simulink model "Simulation_Sprungantwort"  (R2019a)
settings: Solver=FixedStepAuto  StartTime=0.0  StopTime=12  FixedStep=1/1e4  RelTol=1e-3
settings Model: Creator=basti  LastModifiedBy=aaron
settings DebuggingCC: SFMachineParentedDataDiag=error

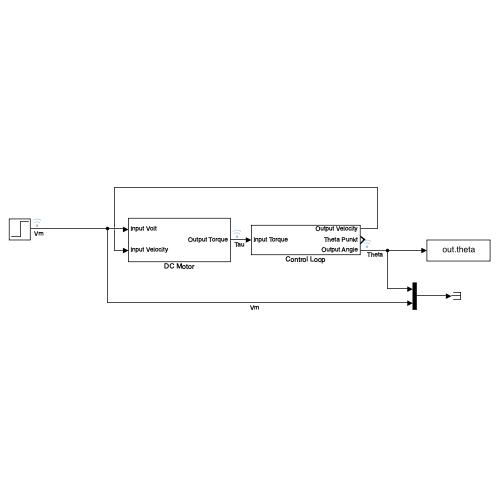
[thumbnail: Simulink's stored preview of the top-level diagram]
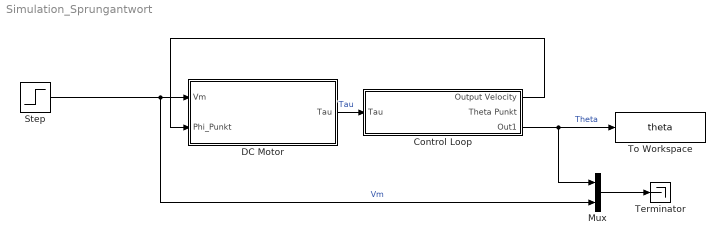
== system Simulation_Sprungantwort ==
  Control Loop : Subsystem
  DC Motor : Subsystem
  Mux : Mux  Inputs=2
  Step : Step  Time=0.5  After=[10 15 20]  SampleTime=0
  Terminator : Terminator
  To Workspace : ToWorkspace  VariableName=theta  SampleTime=-1
  wires:
  DC Motor/1(Tau) -> Control Loop/1(Tau)  "Tau"
  Control Loop/1(Output Velocity) -> DC Motor/2(Phi_Punkt)
  Control Loop/3(Out1) -> To Workspace/1, Mux/1  "Theta"
  Mux/1 -> Terminator/1
  Step/1 -> Mux/2, DC Motor/1(Vm)  "Vm"

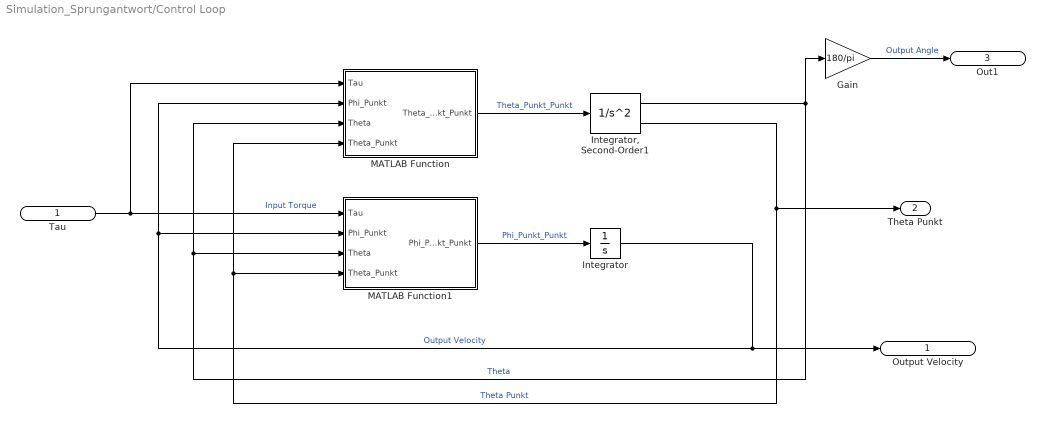
== system Simulation_Sprungantwort/Control Loop ==
  Tau : Inport
  Gain : Gain  Gain=180/pi
  Integrator : Integrator
  "Integrator, Second-Order1" : SecondOrderIntegrator  ICX=pi
  MATLAB Function : MATLAB Function  TreatAsAtomicUnit=on
  MATLAB Function1 : MATLAB Function  TreatAsAtomicUnit=on
  Output Velocity : Outport
  Theta Punkt : Outport  Port=2
  Out1 : Outport  Port=3
  wires:
  MATLAB Function/1(Theta_Punkt_Punkt) -> "Integrator, Second-Order1"/1  "Theta_Punkt_Punkt"
  MATLAB Function1/1(Phi_Punkt_Punkt) -> Integrator/1  "Phi_Punkt_Punkt"
  Integrator/1 -> Output Velocity/1, MATLAB Function1/2(Phi_Punkt), MATLAB Function/2(Phi_Punkt)  "Output Velocity"
  "Integrator, Second-Order1"/1 -> MATLAB Function1/3(Theta), MATLAB Function/3(Theta), Gain/1  "Theta"
  "Integrator, Second-Order1"/2 -> Theta Punkt/1, MATLAB Function/4(Theta_Punkt), MATLAB Function1/4(Theta_Punkt)  "Theta Punkt"
  Tau/1 -> MATLAB Function/1(Tau), MATLAB Function1/1(Tau)  "Input Torque"
  Gain/1 -> Out1/1  "Output Angle"

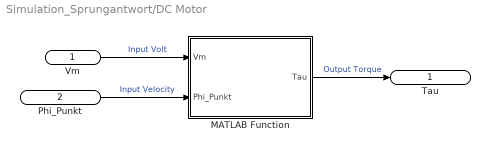
== system Simulation_Sprungantwort/DC Motor ==
  Vm : Inport
  Phi_Punkt : Inport  Port=2
  MATLAB Function : MATLAB Function  TreatAsAtomicUnit=on
  Tau : Outport
  wires:
  Vm/1 -> MATLAB Function/1(Vm)  "Input Volt"
  Phi_Punkt/1 -> MATLAB Function/2(Phi_Punkt)  "Input Velocity"
  MATLAB Function/1(Tau) -> Tau/1  "Output Torque"

== matlab function Simulation_Sprungantwort/Control Loop/MATLAB Function1 ==
  data: Tau input; Phi_Punkt_Punkt output; Phi_Punkt input; Theta input; Theta_Punkt input
function Phi_Punkt_Punkt = fcn(Tau, Phi_Punkt, Theta, Theta_Punkt)
    % Konstanten aufrufen
    c = Konstanten();
    
    % Berechnung
    Phi_Punkt_Punkt = (((c.m1*c.l1+c.m2*c.l2)*c.g*sin(Theta)-c.c1*Theta_Punkt-(c.m1*c.l1^2+c.m2*c.l2^2+c.J1+c.J2)*(Tau-c.c2*Phi_Punkt)/c.J2)/c.J2)/(1-(c.m1*c.l1^2+c.m2*c.l2^2+c.J1+c.J2)/c.J2);

== matlab function Simulation_Sprungantwort/Control Loop/MATLAB Function ==
  data: Tau input; Theta_Punkt_Punkt output; Phi_Punkt input; Theta input; Theta_Punkt input
function Theta_Punkt_Punkt = fcn(Tau, Phi_Punkt, Theta, Theta_Punkt)
    % Konstanten aufrufen
    c = Konstanten();
    
    % Berechnung
    Theta_Punkt_Punkt = ((Tau-c.c2*Phi_Punkt-(c.m1*c.l1+c.m2*c.l2)*c.g*sin(Theta)+c.c1*Theta_Punkt)/c.J2)/(1-(c.m1*c.l1^2+c.m2*c.l2^2+c.J1+c.J2)/c.J2);

== matlab function Simulation_Sprungantwort/DC Motor/MATLAB Function ==
  data: Vm input; Tau output; Phi_Punkt input
function Tau = fcn(Vm, Phi_Punkt)
    % Konstanten
    c = Konstanten();
    
    % Berechnung
    Tau = c.Kt*(Vm-c.Kb*Phi_Punkt)/c.Ra;
